simulink model "ch423"  (Simulink 8.1)
settings: Solver=ode45  StartTime=0.0  StopTime=20  RelTol=1e-3
settings Model: Creator=jmahler  LastModifiedBy=jmahler
settings DataIOCC: SignalLoggingSaveFormat=Dataset
settings OptimizationCC: ExpressionDepthLimit=128
settings DebuggingCC: FcnCallInpInsideContextMsg=EnableAllAsError
settings GRTTargetCC: CombineOutputUpdateFcns=on  GRTInterface=off

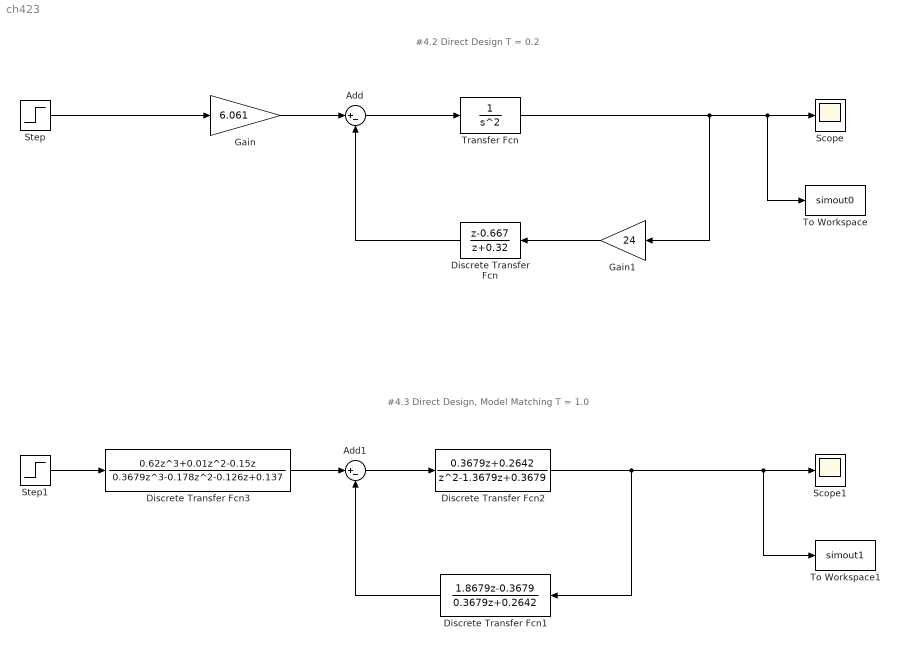
== system ch423 ==
  note: #4.2  Direct Design
      | T = 0.2
  note: #4.3  Direct Design, Model Matching
      | T = 1.0
  Add : Sum  Inputs=|+-
  Add1 : Sum  Inputs=|+-
  Discrete Transfer Fcn : DiscreteTransferFcn  Numerator=[1 -0.667]  Denominator=[1 0.32]  SampleTime=0.2
  Discrete Transfer Fcn1 : DiscreteTransferFcn  Numerator=[1.8679 -0.3679]  Denominator=[0.3679 0.2642]  SampleTime=1
  Discrete Transfer Fcn2 : DiscreteTransferFcn  Numerator=[0.3679 0.2642]  Denominator=[1 -1.3679 0.3679]  SampleTime=1
  Discrete Transfer Fcn3 : DiscreteTransferFcn  Numerator=[0.62 0.01 -0.15 0]  Denominator=[0.3679 -0.178 -0.126 0.137]  SampleTime=1
  Gain : Gain  Gain=6.061
  Gain1 : Gain  Gain=24
  Scope : Scope
  Scope1 : Scope
  Step : Step  Time=0  SampleTime=0
  Step1 : Step  Time=0  SampleTime=0
  To Workspace : ToWorkspace  VariableName=simout0  SampleTime=-1  SaveFormat=Timeseries
  To Workspace1 : ToWorkspace  VariableName=simout1  SampleTime=-1  SaveFormat=Timeseries
  Transfer Fcn : TransferFcn  Denominator=[1 0 0]
  wires:
  Gain1/1 -> Discrete Transfer Fcn/1
  Transfer Fcn/1 -> Gain1/1, To Workspace/1, Scope/1
  Discrete Transfer Fcn/1 -> Add/2
  Add/1 -> Transfer Fcn/1
  Gain/1 -> Add/1
  Step/1 -> Gain/1
  Discrete Transfer Fcn1/1 -> Add1/2
  Add1/1 -> Discrete Transfer Fcn2/1
  Discrete Transfer Fcn2/1 -> Discrete Transfer Fcn1/1, To Workspace1/1, Scope1/1
  Step1/1 -> Discrete Transfer Fcn3/1
  Discrete Transfer Fcn3/1 -> Add1/1
